simulink model "MAS_pc_up"  (R2022b)
settings: Solver=VariableStepAuto  StartTime=0.0  StopTime=300  RelTol=1e-3
values from neighbouring files (symbols this model uses):
  a1 = int8(3)    [init.m]
  A1 = [1.7,-1.3 ... (first row only)    [init.m]
  A2 = [1.8,-1.4 ... (first row only)    [init.m]
  a2 = int8(2)    [init.m]
  A3 = [1.4,-1.1 ... (first row only)    [init.m]
  a3 = int8(3)    [init.m]
  B1 = [1.0 ... (first row only)    [init.m]
  B2 = [1.7 ... (first row only)    [init.m]
  B3 = [0.8 ... (first row only)    [init.m]
  C1 = [1.0,0.3]    [init.m]
  C2 = [0.7,0.2]    [init.m]
  C3 = [1.1,0.4]    [init.m]
  F1 = [-0.4483 ... (first row only)    [init.m]
  F2 = [-0.6803 ... (first row only)    [init.m]
  F3 = [-0.3908 ... (first row only)    [init.m]
  G1 = -0.16    [init.m]
  G2 = -0.18    [init.m]
  G3 = -0.14    [init.m]
  H1 = -0.12    [init.m]
  H2 = -0.10    (= -0.1)    [init.m]
  H3 = -0.14    [init.m]
  M = [1,0,1 ... (first row only)    [init.m]
  s1 = int8(2)    [init.m]
  s2 = int8(3)    [init.m]
  s3 = int8(1)    [init.m]
  samp_t = 0.2    [init.m]
(part 2 of 2)

== system MAS_pc_up/u7 ==
  z : Inport
  hat_Y : Inport  Port=2
  Add : Sum
  Constant1 : Constant  Value=M
  Constant2 : Constant  Value=id
  G : Constant  Value=G1  VectorParams1D=off
  H : Constant  Value=H1  VectorParams1D=off
  MATLAB Function : MATLAB Function  TreatAsAtomicUnit=on
  Product : Product  Multiplication=Matrix(*)
  Product1 : Product  Multiplication=Matrix(*)
  u : Outport
  wires:
  z/1 -> Product/2
  G/1 -> Product/1
  Product/1 -> Add/1
  Add/1 -> u/1
  Constant1/1 -> MATLAB Function/1(M)
  hat_Y/1 -> MATLAB Function/2(hat_Y)
  Constant2/1 -> MATLAB Function/3(id)
  MATLAB Function/1(y) -> Product1/2
  H/1 -> Product1/1
  Product1/1 -> Add/2

== system MAS_pc_up/u8 ==
  z : Inport
  hat_Y : Inport  Port=2
  Add : Sum
  Constant1 : Constant  Value=M
  Constant2 : Constant  Value=id
  G : Constant  Value=G2  VectorParams1D=off
  H : Constant  Value=H2  VectorParams1D=off
  MATLAB Function : MATLAB Function  TreatAsAtomicUnit=on
  Product : Product  Multiplication=Matrix(*)
  Product1 : Product  Multiplication=Matrix(*)
  u : Outport
  wires:
  z/1 -> Product/2
  G/1 -> Product/1
  Product/1 -> Add/1
  Add/1 -> u/1
  Constant1/1 -> MATLAB Function/1(M)
  hat_Y/1 -> MATLAB Function/2(hat_Y)
  Constant2/1 -> MATLAB Function/3(id)
  MATLAB Function/1(y) -> Product1/2
  H/1 -> Product1/1
  Product1/1 -> Add/2

== system MAS_pc_up/u9 ==
  z : Inport
  hat_Y : Inport  Port=2
  Add : Sum
  Constant1 : Constant  Value=M
  Constant2 : Constant  Value=id
  G : Constant  Value=G3  VectorParams1D=off
  H : Constant  Value=H3  VectorParams1D=off
  MATLAB Function : MATLAB Function  TreatAsAtomicUnit=on
  Product : Product  Multiplication=Matrix(*)
  Product1 : Product  Multiplication=Matrix(*)
  u : Outport
  wires:
  z/1 -> Product/2
  G/1 -> Product/1
  Product/1 -> Add/1
  Add/1 -> u/1
  Constant1/1 -> MATLAB Function/1(M)
  hat_Y/1 -> MATLAB Function/2(hat_Y)
  Constant2/1 -> MATLAB Function/3(id)
  MATLAB Function/1(y) -> Product1/2
  H/1 -> Product1/1
  Product1/1 -> Add/2

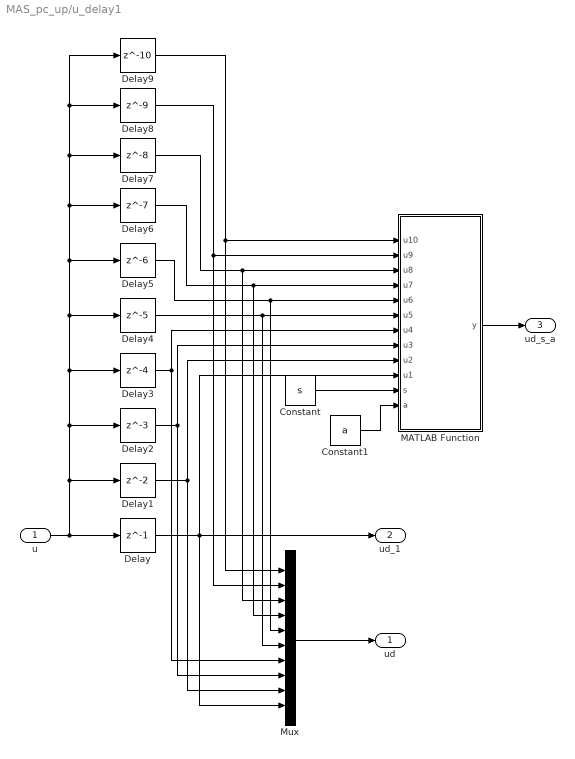
== system MAS_pc_up/u_delay1 ==
  u : Inport
  Constant : Constant  Value=s
  Constant1 : Constant  Value=a
  Delay : Delay  DelayLength=1  InitialCondition=0  SampleTime=samp_t
  Delay1 : Delay  InitialCondition=0  SampleTime=samp_t
  Delay2 : Delay  DelayLength=3  InitialCondition=0  SampleTime=samp_t
  Delay3 : Delay  DelayLength=4  InitialCondition=0  SampleTime=samp_t
  Delay4 : Delay  DelayLength=5  InitialCondition=0  SampleTime=samp_t
  Delay5 : Delay  DelayLength=6  InitialCondition=0  SampleTime=samp_t
  Delay6 : Delay  DelayLength=7  InitialCondition=0  SampleTime=samp_t
  Delay7 : Delay  DelayLength=8  InitialCondition=0  SampleTime=samp_t
  Delay8 : Delay  DelayLength=9  InitialCondition=0  SampleTime=samp_t
  Delay9 : Delay  DelayLength=10  InitialCondition=0  SampleTime=samp_t
  MATLAB Function : MATLAB Function  TreatAsAtomicUnit=on
  Mux : Mux  Inputs=10
  ud : Outport
  ud_1 : Outport  Port=2
  ud_s_a : Outport  Port=3
  wires:
  u/1 -> Delay/1, Delay1/1, Delay2/1, Delay3/1, Delay4/1, Delay6/1, Delay7/1, Delay8/1, Delay9/1, Delay5/1
  Delay/1 -> Mux/10, MATLAB Function/10(u1), ud_1/1
  Delay4/1 -> MATLAB Function/6(u5), Mux/6
  Delay3/1 -> Mux/7, MATLAB Function/7(u4)
  Delay2/1 -> Mux/8, MATLAB Function/8(u3)
  Delay1/1 -> Mux/9, MATLAB Function/9(u2)
  MATLAB Function/1(y) -> ud_s_a/1
  Mux/1 -> ud/1
  Delay5/1 -> Mux/5, MATLAB Function/5(u6)
  Delay6/1 -> MATLAB Function/4(u7), Mux/4
  Delay7/1 -> MATLAB Function/3(u8), Mux/3
  Delay8/1 -> MATLAB Function/2(u9), Mux/2
  Delay9/1 -> MATLAB Function/1(u10), Mux/1
  Constant/1 -> MATLAB Function/11(s)
  Constant1/1 -> MATLAB Function/12(a)

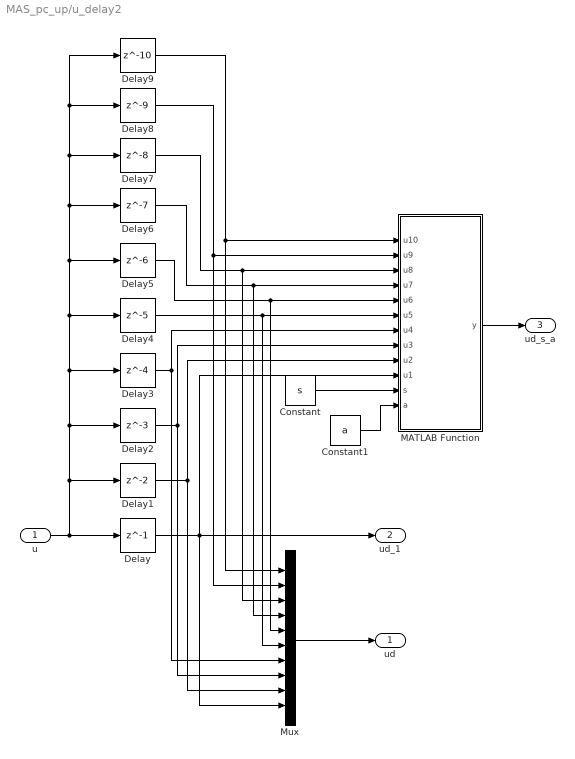
== system MAS_pc_up/u_delay2 ==
  u : Inport
  Constant : Constant  Value=s
  Constant1 : Constant  Value=a
  Delay : Delay  DelayLength=1  InitialCondition=0  SampleTime=samp_t
  Delay1 : Delay  InitialCondition=0  SampleTime=samp_t
  Delay2 : Delay  DelayLength=3  InitialCondition=0  SampleTime=samp_t
  Delay3 : Delay  DelayLength=4  InitialCondition=0  SampleTime=samp_t
  Delay4 : Delay  DelayLength=5  InitialCondition=0  SampleTime=samp_t
  Delay5 : Delay  DelayLength=6  InitialCondition=0  SampleTime=samp_t
  Delay6 : Delay  DelayLength=7  InitialCondition=0  SampleTime=samp_t
  Delay7 : Delay  DelayLength=8  InitialCondition=0  SampleTime=samp_t
  Delay8 : Delay  DelayLength=9  InitialCondition=0  SampleTime=samp_t
  Delay9 : Delay  DelayLength=10  InitialCondition=0  SampleTime=samp_t
  MATLAB Function : MATLAB Function  TreatAsAtomicUnit=on
  Mux : Mux  Inputs=10
  ud : Outport
  ud_1 : Outport  Port=2
  ud_s_a : Outport  Port=3
  wires:
  u/1 -> Delay/1, Delay1/1, Delay2/1, Delay3/1, Delay4/1, Delay6/1, Delay7/1, Delay8/1, Delay9/1, Delay5/1
  Delay/1 -> Mux/10, MATLAB Function/10(u1), ud_1/1
  Delay4/1 -> MATLAB Function/6(u5), Mux/6
  Delay3/1 -> Mux/7, MATLAB Function/7(u4)
  Delay2/1 -> Mux/8, MATLAB Function/8(u3)
  Delay1/1 -> Mux/9, MATLAB Function/9(u2)
  MATLAB Function/1(y) -> ud_s_a/1
  Mux/1 -> ud/1
  Delay5/1 -> Mux/5, MATLAB Function/5(u6)
  Delay6/1 -> MATLAB Function/4(u7), Mux/4
  Delay7/1 -> MATLAB Function/3(u8), Mux/3
  Delay8/1 -> MATLAB Function/2(u9), Mux/2
  Delay9/1 -> MATLAB Function/1(u10), Mux/1
  Constant/1 -> MATLAB Function/11(s)
  Constant1/1 -> MATLAB Function/12(a)

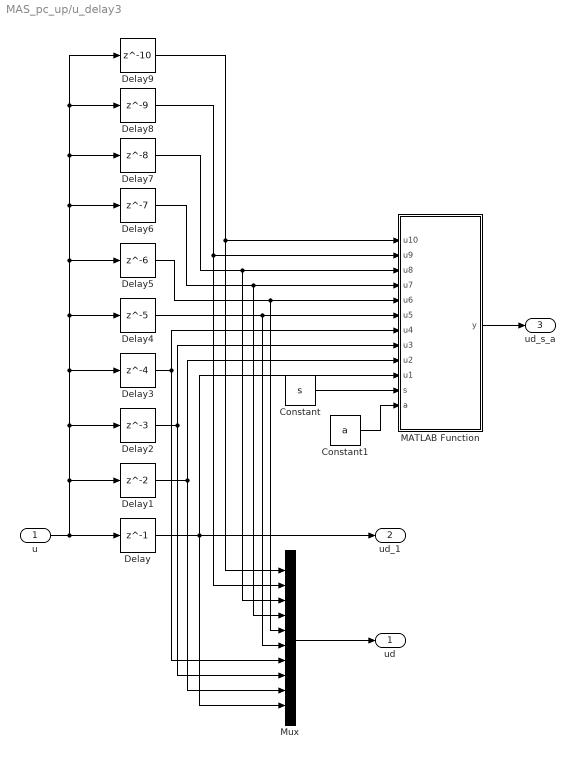
== system MAS_pc_up/u_delay3 ==
  u : Inport
  Constant : Constant  Value=s
  Constant1 : Constant  Value=a
  Delay : Delay  DelayLength=1  InitialCondition=0  SampleTime=samp_t
  Delay1 : Delay  InitialCondition=0  SampleTime=samp_t
  Delay2 : Delay  DelayLength=3  InitialCondition=0  SampleTime=samp_t
  Delay3 : Delay  DelayLength=4  InitialCondition=0  SampleTime=samp_t
  Delay4 : Delay  DelayLength=5  InitialCondition=0  SampleTime=samp_t
  Delay5 : Delay  DelayLength=6  InitialCondition=0  SampleTime=samp_t
  Delay6 : Delay  DelayLength=7  InitialCondition=0  SampleTime=samp_t
  Delay7 : Delay  DelayLength=8  InitialCondition=0  SampleTime=samp_t
  Delay8 : Delay  DelayLength=9  InitialCondition=0  SampleTime=samp_t
  Delay9 : Delay  DelayLength=10  InitialCondition=0  SampleTime=samp_t
  MATLAB Function : MATLAB Function  TreatAsAtomicUnit=on
  Mux : Mux  Inputs=10
  ud : Outport
  ud_1 : Outport  Port=2
  ud_s_a : Outport  Port=3
  wires:
  u/1 -> Delay/1, Delay1/1, Delay2/1, Delay3/1, Delay4/1, Delay6/1, Delay7/1, Delay8/1, Delay9/1, Delay5/1
  Delay/1 -> Mux/10, MATLAB Function/10(u1), ud_1/1
  Delay4/1 -> MATLAB Function/6(u5), Mux/6
  Delay3/1 -> Mux/7, MATLAB Function/7(u4)
  Delay2/1 -> Mux/8, MATLAB Function/8(u3)
  Delay1/1 -> Mux/9, MATLAB Function/9(u2)
  MATLAB Function/1(y) -> ud_s_a/1
  Mux/1 -> ud/1
  Delay5/1 -> Mux/5, MATLAB Function/5(u6)
  Delay6/1 -> MATLAB Function/4(u7), Mux/4
  Delay7/1 -> MATLAB Function/3(u8), Mux/3
  Delay8/1 -> MATLAB Function/2(u9), Mux/2
  Delay9/1 -> MATLAB Function/1(u10), Mux/1
  Constant/1 -> MATLAB Function/11(s)
  Constant1/1 -> MATLAB Function/12(a)

== system MAS_pc_up/u_delay4 ==
  u : Inport
  Constant : Constant  Value=s
  Delay : Delay  DelayLength=1  InitialCondition=0  SampleTime=samp_t
  Delay1 : Delay  InitialCondition=0  SampleTime=samp_t
  Delay2 : Delay  DelayLength=3  InitialCondition=0  SampleTime=samp_t
  Delay3 : Delay  DelayLength=4  InitialCondition=0  SampleTime=samp_t
  Delay4 : Delay  DelayLength=5  InitialCondition=0  SampleTime=samp_t
  MATLAB Function : MATLAB Function  TreatAsAtomicUnit=on
  Mux : Mux  Inputs=5
  ud : Outport
  ud_1 : Outport  Port=2
  ud_s : Outport  Port=3
  wires:
  u/1 -> Delay/1, Delay1/1, Delay2/1, Delay3/1, Delay4/1
  Delay/1 -> ud_1/1, MATLAB Function/6(u1), Mux/5
  Constant/1 -> MATLAB Function/1(s)
  Delay4/1 -> Mux/1, MATLAB Function/2(u5)
  Delay3/1 -> Mux/2, MATLAB Function/3(u4)
  Delay2/1 -> Mux/3, MATLAB Function/4(u3)
  Delay1/1 -> Mux/4, MATLAB Function/5(u2)
  MATLAB Function/1(y) -> ud_s/1
  Mux/1 -> ud/1

== system MAS_pc_up/u_delay5 ==
  u : Inport
  Constant : Constant  Value=s  OutDataTypeStr=int64
  Delay : Delay  DelayLength=1  InitialCondition=0  SampleTime=samp_t
  Delay1 : Delay  InitialCondition=0  SampleTime=samp_t
  Delay2 : Delay  DelayLength=3  InitialCondition=0  SampleTime=samp_t
  Delay3 : Delay  DelayLength=4  InitialCondition=0  SampleTime=samp_t
  Delay4 : Delay  DelayLength=5  InitialCondition=0  SampleTime=samp_t
  MATLAB Function : MATLAB Function  TreatAsAtomicUnit=on
  Mux : Mux  Inputs=5
  ud : Outport
  ud_1 : Outport  Port=2
  ud_s : Outport  Port=3
  wires:
  u/1 -> Delay/1, Delay1/1, Delay2/1, Delay3/1, Delay4/1
  Delay/1 -> ud_1/1, MATLAB Function/6(u1), Mux/5
  Constant/1 -> MATLAB Function/1(s)
  Delay4/1 -> Mux/1, MATLAB Function/2(u5)
  Delay3/1 -> Mux/2, MATLAB Function/3(u4)
  Delay2/1 -> Mux/3, MATLAB Function/4(u3)
  Delay1/1 -> Mux/4, MATLAB Function/5(u2)
  MATLAB Function/1(y) -> ud_s/1
  Mux/1 -> ud/1

== system MAS_pc_up/u_delay6 ==
  u : Inport
  Constant : Constant  Value=s
  Delay : Delay  DelayLength=1  InitialCondition=0  SampleTime=samp_t
  Delay1 : Delay  InitialCondition=0  SampleTime=samp_t
  Delay2 : Delay  DelayLength=3  InitialCondition=0  SampleTime=samp_t
  Delay3 : Delay  DelayLength=4  InitialCondition=0  SampleTime=samp_t
  Delay4 : Delay  DelayLength=5  InitialCondition=0  SampleTime=samp_t
  MATLAB Function : MATLAB Function  TreatAsAtomicUnit=on
  Mux : Mux  Inputs=5
  ud : Outport
  ud_1 : Outport  Port=2
  ud_s : Outport  Port=3
  wires:
  u/1 -> Delay/1, Delay1/1, Delay2/1, Delay3/1, Delay4/1
  Delay/1 -> ud_1/1, MATLAB Function/6(u1), Mux/5
  Constant/1 -> MATLAB Function/1(s)
  Delay4/1 -> Mux/1, MATLAB Function/2(u5)
  Delay3/1 -> Mux/2, MATLAB Function/3(u4)
  Delay2/1 -> Mux/3, MATLAB Function/4(u3)
  Delay1/1 -> Mux/4, MATLAB Function/5(u2)
  MATLAB Function/1(y) -> ud_s/1
  Mux/1 -> ud/1

== matlab function MAS_pc_up/u2/MATLAB Function ==
  data: M input; y output; hat_Y input; id input
function y = fcn(M,hat_Y,id)
y = zeros(size(hat_Y(id,:)))
for i = 1:length(M(id,:))
    if M(id,i)==1
        y = y + hat_Y(i,:) - hat_Y(id,:)
    end

end

== matlab function MAS_pc_up/u3/MATLAB Function ==
  data: M input; y output; hat_Y input; id input
function y = fcn(M,hat_Y,id)
y = zeros(size(hat_Y(id,:)))
for i = 1:length(M(id,:))
    if M(id,i)==1
        y = y + hat_Y(i,:) - hat_Y(id,:)
    end

end

== matlab function MAS_pc_up/u_delay1/MATLAB Function ==
  data: u10 input; u9 input; u8 input; u7 input; u6 input; y output size=1*1; u5 input size=1*1; u4 input size=1*1; u3 input size=1*1; u2 input size=1*1; u1 input size=1*1; s input; a input
function y = fcn(u10,u9,u8,u7,u6,u5,u4,u3,u2,u1,s,a)
tmp = s + a;
if tmp==1
    y = u1;
elseif tmp==2
    y = u2;
elseif tmp==3
    y = u3;
elseif tmp==4
    y = u4;
elseif tmp==5
    y = u5;
elseif tmp==6
    y = u6;
elseif tmp==7
    y = u7;
elseif tmp==8
    y = u8;
elseif tmp==9
    y = u9;
elseif tmp==10
    y = u10;
else
    y = u1
disp("mmp_error")
end

== matlab function MAS_pc_up/u_delay2/MATLAB Function ==
  data: u10 input; u9 input; u8 input; u7 input; u6 input; y output size=1*1; u5 input size=1*1; u4 input size=1*1; u3 input size=1*1; u2 input size=1*1; u1 input size=1*1; s input; a input
function y = fcn(u10,u9,u8,u7,u6,u5,u4,u3,u2,u1,s,a)
tmp = s + a;
if tmp==1
    y = u1;
elseif tmp==2
    y = u2;
elseif tmp==3
    y = u3;
elseif tmp==4
    y = u4;
elseif tmp==5
    y = u5;
elseif tmp==6
    y = u6;
elseif tmp==7
    y = u7;
elseif tmp==8
    y = u8;
elseif tmp==9
    y = u9;
elseif tmp==10
    y = u10;
else
    y = u1
disp("mmp_error")
end

== matlab function MAS_pc_up/u_delay3/MATLAB Function ==
  data: u10 input; u9 input; u8 input; u7 input; u6 input; y output size=1*1; u5 input size=1*1; u4 input size=1*1; u3 input size=1*1; u2 input size=1*1; u1 input size=1*1; s input; a input
function y = fcn(u10,u9,u8,u7,u6,u5,u4,u3,u2,u1,s,a)
tmp = s + a;
if tmp==1
    y = u1;
elseif tmp==2
    y = u2;
elseif tmp==3
    y = u3;
elseif tmp==4
    y = u4;
elseif tmp==5
    y = u5;
elseif tmp==6
    y = u6;
elseif tmp==7
    y = u7;
elseif tmp==8
    y = u8;
elseif tmp==9
    y = u9;
elseif tmp==10
    y = u10;
else
    y = u1
disp("mmp_error")
end

== matlab function MAS_pc_up/Ps2a2/MATLAB Function ==
  data: u10 input; u9 input; u8 input; u7 input; u6 input; x_ output size=2*1; u5 input; u4 input; u3 input; u2 input; u1 input; y output size=1*1; x input size=2*1; s input; a input; A input; B input; C input
function [x_,y]= fcn(u10,u9,u8,u7,u6,u5,u4,u3,u2,u1,x,s,a,A,B,C)
% tau的上界是N,最多迭代N次，控制输入按照t-s_i时刻的值
tau = s + a;
temp0 = x;
if tau == 1
    temp1 = A * temp0 + B * u1;
    x_ = temp1;
elseif tau == 2
    temp1 = A * temp0 + B * u2;
    temp2 = A * temp1 + B * u1;
    x_ = temp2;
elseif tau == 3
    temp1 = A * temp0 + B * u3;
    temp2 = A * temp1 + B * u2;
    temp3 = A * temp2 + B * u1;
    x_ = temp3;
elseif tau == 4
    temp1 = A * temp0 + B * u4;
    temp2 = A * temp1 + B * u3;
    temp3 = A * temp2 + B * u2;
    temp4 = A * temp3 + B * u1;
    x_ = temp4;  
elseif tau == 5
    temp1 = A * temp0 + B * u5;
    temp2 = A * temp1 + B * u4;
    temp3 = A * temp2 + B * u3;
    temp4 = A * temp3 + B * u2;
    temp5 = A * temp4 + B * u1;
    x_ = temp5;
elseif tau == 6
    temp1 = A * temp0 + B * u6;
    temp2 = A * temp1 + B * u5;
    temp3 = A * temp2 + B * u4;
    temp4 = A * temp3 + B * u3;
    temp5 = A * temp4 + B * u2;
    temp6 = A * temp5 + B * u1;
    x_ = temp6;
elseif tau == 7
    temp1 = A * temp0 + B * u7;
    temp2 = A * temp1 + B * u6;
    temp3 = A * temp2 + B * u5;
    temp4 = A * temp3 + B * u4;
    temp5 = A * temp4 + B * u3;
    temp6 = A * temp5 + B * u2;
    temp7 = A * temp6 + B * u2;
    x_ = temp7;
elseif tau == 8
    temp1 = A * temp0 + B * u8;
    temp2 = A * temp1 + B * u7;
    temp3 = A * temp2 + B * u6;
    temp4 = A * temp3 + B * u5;
    temp5 = A * temp4 + B * u4;
    temp6 = A * temp5 + B * u3;
    temp7 = A * temp6 + B * u2;
    temp8 = A * temp7 + B * u1;
    x_ = temp8;
elseif tau == 9
    temp1 = A * temp0 + B * u9;
    temp2 = A * temp1 + B * u8;
    temp3 = A * temp2 + B * u7;
    temp4 = A * temp3 + B * u6;
    temp5 = A * temp4 + B * u5;
    temp6 = A * temp5 + B * u4;
    temp7 = A * temp6 + B * u3;
    temp8 = A * temp7 + B * u2;
    temp9 = A * temp8 + B * u1;
    x_ = temp9;
elseif tau == 10
    temp1 = A * temp0 + B * u10;
    temp2 = A * temp1 + B * u9;
    temp3 = A * temp2 + B * u8;
    temp4 = A * temp3 + B * u7;
    temp5 = A * temp4 + B * u6;
    temp6 = A * temp5 + B * u5;
    temp7 = A * temp6 + B * u4;
    temp8 = A * temp7 + B * u3;
    temp9 = A * temp8 + B * u2;
    temp10 = A * temp9 + B * u1;
    x_ = temp10;
else 
    x_ = temp0;

end
y = C * x_;

== matlab function MAS_pc_up/Ps2a1/MATLAB Function ==
  data: u10 input; u9 input; u8 input; u7 input; u6 input; x_ output size=2*1; u5 input; u4 input; u3 input; u2 input; u1 input; y output size=1*1; x input size=2*1; s input; a input; A input; B input; C input
function [x_,y]= fcn(u10,u9,u8,u7,u6,u5,u4,u3,u2,u1,x,s,a,A,B,C)
% tau的上界是N,最多迭代N次，控制输入按照t-s_i时刻的值
tau = s + a;
temp0 = x;
if tau == 1
    temp1 = A * temp0 + B * u1;
    x_ = temp1;
elseif tau == 2
    temp1 = A * temp0 + B * u2;
    temp2 = A * temp1 + B * u1;
    x_ = temp2;
elseif tau == 3
    temp1 = A * temp0 + B * u3;
    temp2 = A * temp1 + B * u2;
    temp3 = A * temp2 + B * u1;
    x_ = temp3;
elseif tau == 4
    temp1 = A * temp0 + B * u4;
    temp2 = A * temp1 + B * u3;
    temp3 = A * temp2 + B * u2;
    temp4 = A * temp3 + B * u1;
    x_ = temp4;  
elseif tau == 5
    temp1 = A * temp0 + B * u5;
    temp2 = A * temp1 + B * u4;
    temp3 = A * temp2 + B * u3;
    temp4 = A * temp3 + B * u2;
    temp5 = A * temp4 + B * u1;
    x_ = temp5;
elseif tau == 6
    temp1 = A * temp0 + B * u6;
    temp2 = A * temp1 + B * u5;
    temp3 = A * temp2 + B * u4;
    temp4 = A * temp3 + B * u3;
    temp5 = A * temp4 + B * u2;
    temp6 = A * temp5 + B * u1;
    x_ = temp6;
elseif tau == 7
    temp1 = A * temp0 + B * u7;
    temp2 = A * temp1 + B * u6;
    temp3 = A * temp2 + B * u5;
    temp4 = A * temp3 + B * u4;
    temp5 = A * temp4 + B * u3;
    temp6 = A * temp5 + B * u2;
    temp7 = A * temp6 + B * u2;
    x_ = temp7;
elseif tau == 8
    temp1 = A * temp0 + B * u8;
    temp2 = A * temp1 + B * u7;
    temp3 = A * temp2 + B * u6;
    temp4 = A * temp3 + B * u5;
    temp5 = A * temp4 + B * u4;
    temp6 = A * temp5 + B * u3;
    temp7 = A * temp6 + B * u2;
    temp8 = A * temp7 + B * u1;
    x_ = temp8;
elseif tau == 9
    temp1 = A * temp0 + B * u9;
    temp2 = A * temp1 + B * u8;
    temp3 = A * temp2 + B * u7;
    temp4 = A * temp3 + B * u6;
    temp5 = A * temp4 + B * u5;
    temp6 = A * temp5 + B * u4;
    temp7 = A * temp6 + B * u3;
    temp8 = A * temp7 + B * u2;
    temp9 = A * temp8 + B * u1;
    x_ = temp9;
elseif tau == 10
    temp1 = A * temp0 + B * u10;
    temp2 = A * temp1 + B * u9;
    temp3 = A * temp2 + B * u8;
    temp4 = A * temp3 + B * u7;
    temp5 = A * temp4 + B * u6;
    temp6 = A * temp5 + B * u5;
    temp7 = A * temp6 + B * u4;
    temp8 = A * temp7 + B * u3;
    temp9 = A * temp8 + B * u2;
    temp10 = A * temp9 + B * u1;
    x_ = temp10;
else 
    x_ = temp0;

end
y = C * x_;

== matlab function MAS_pc_up/Ps2a3/MATLAB Function ==
  data: u10 input; u9 input; u8 input; u7 input; u6 input; x_ output size=2*1; u5 input; u4 input; u3 input; u2 input; u1 input; y output size=1*1; x input size=2*1; s input; a input; A input; B input; C input
function [x_,y]= fcn(u10,u9,u8,u7,u6,u5,u4,u3,u2,u1,x,s,a,A,B,C)
% tau的上界是N,最多迭代N次，控制输入按照t-s_i时刻的值
tau = s + a;
temp0 = x;
if tau == 1
    temp1 = A * temp0 + B * u1;
    x_ = temp1;
elseif tau == 2
    temp1 = A * temp0 + B * u2;
    temp2 = A * temp1 + B * u1;
    x_ = temp2;
elseif tau == 3
    temp1 = A * temp0 + B * u3;
    temp2 = A * temp1 + B * u2;
    temp3 = A * temp2 + B * u1;
    x_ = temp3;
elseif tau == 4
    temp1 = A * temp0 + B * u4;
    temp2 = A * temp1 + B * u3;
    temp3 = A * temp2 + B * u2;
    temp4 = A * temp3 + B * u1;
    x_ = temp4;  
elseif tau == 5
    temp1 = A * temp0 + B * u5;
    temp2 = A * temp1 + B * u4;
    temp3 = A * temp2 + B * u3;
    temp4 = A * temp3 + B * u2;
    temp5 = A * temp4 + B * u1;
    x_ = temp5;
elseif tau == 6
    temp1 = A * temp0 + B * u6;
    temp2 = A * temp1 + B * u5;
    temp3 = A * temp2 + B * u4;
    temp4 = A * temp3 + B * u3;
    temp5 = A * temp4 + B * u2;
    temp6 = A * temp5 + B * u1;
    x_ = temp6;
elseif tau == 7
    temp1 = A * temp0 + B * u7;
    temp2 = A * temp1 + B * u6;
    temp3 = A * temp2 + B * u5;
    temp4 = A * temp3 + B * u4;
    temp5 = A * temp4 + B * u3;
    temp6 = A * temp5 + B * u2;
    temp7 = A * temp6 + B * u2;
    x_ = temp7;
elseif tau == 8
    temp1 = A * temp0 + B * u8;
    temp2 = A * temp1 + B * u7;
    temp3 = A * temp2 + B * u6;
    temp4 = A * temp3 + B * u5;
    temp5 = A * temp4 + B * u4;
    temp6 = A * temp5 + B * u3;
    temp7 = A * temp6 + B * u2;
    temp8 = A * temp7 + B * u1;
    x_ = temp8;
elseif tau == 9
    temp1 = A * temp0 + B * u9;
    temp2 = A * temp1 + B * u8;
    temp3 = A * temp2 + B * u7;
    temp4 = A * temp3 + B * u6;
    temp5 = A * temp4 + B * u5;
    temp6 = A * temp5 + B * u4;
    temp7 = A * temp6 + B * u3;
    temp8 = A * temp7 + B * u2;
    temp9 = A * temp8 + B * u1;
    x_ = temp9;
elseif tau == 10
    temp1 = A * temp0 + B * u10;
    temp2 = A * temp1 + B * u9;
    temp3 = A * temp2 + B * u8;
    temp4 = A * temp3 + B * u7;
    temp5 = A * temp4 + B * u6;
    temp6 = A * temp5 + B * u5;
    temp7 = A * temp6 + B * u4;
    temp8 = A * temp7 + B * u3;
    temp9 = A * temp8 + B * u2;
    temp10 = A * temp9 + B * u1;
    x_ = temp10;
else 
    x_ = temp0;

end
y = C * x_;

== matlab function MAS_pc_up/MATLAB Function2 ==
  data: t input; r output
function r = fcn(t)
if t<100
    r = 1;
elseif t<200
    r = 0;

elseif t<300
    r = 1;
else 
    r = 0;

end

== matlab function MAS_pc_up/Ps3a3/MATLAB Function ==
  data: u10 input; u9 input; u8 input; u7 input; u6 input; x_ output size=2*1; u5 input; u4 input; u3 input; u2 input; u1 input; y output size=1*1; x input size=2*1; s input; a input; A input; B input; C input
function [x_,y]= fcn(u10,u9,u8,u7,u6,u5,u4,u3,u2,u1,x,s,a,A,B,C)
% tau的上界是N,最多迭代N次，控制输入按照t-s_i时刻的值
tau = s + a;
temp0 = x;
if tau == 1
    temp1 = A * temp0 + B * u1;
    x_ = temp1;
elseif tau == 2
    temp1 = A * temp0 + B * u2;
    temp2 = A * temp1 + B * u1;
    x_ = temp2;
elseif tau == 3
    temp1 = A * temp0 + B * u3;
    temp2 = A * temp1 + B * u2;
    temp3 = A * temp2 + B * u1;
    x_ = temp3;
elseif tau == 4
    temp1 = A * temp0 + B * u4;
    temp2 = A * temp1 + B * u3;
    temp3 = A * temp2 + B * u2;
    temp4 = A * temp3 + B * u1;
    x_ = temp4;  
elseif tau == 5
    temp1 = A * temp0 + B * u5;
    temp2 = A * temp1 + B * u4;
    temp3 = A * temp2 + B * u3;
    temp4 = A * temp3 + B * u2;
    temp5 = A * temp4 + B * u1;
    x_ = temp5;
elseif tau == 6
    temp1 = A * temp0 + B * u6;
    temp2 = A * temp1 + B * u5;
    temp3 = A * temp2 + B * u4;
    temp4 = A * temp3 + B * u3;
    temp5 = A * temp4 + B * u2;
    temp6 = A * temp5 + B * u1;
    x_ = temp6;
elseif tau == 7
    temp1 = A * temp0 + B * u7;
    temp2 = A * temp1 + B * u6;
    temp3 = A * temp2 + B * u5;
    temp4 = A * temp3 + B * u4;
    temp5 = A * temp4 + B * u3;
    temp6 = A * temp5 + B * u2;
    temp7 = A * temp6 + B * u2;
    x_ = temp7;
elseif tau == 8
    temp1 = A * temp0 + B * u8;
    temp2 = A * temp1 + B * u7;
    temp3 = A * temp2 + B * u6;
    temp4 = A * temp3 + B * u5;
    temp5 = A * temp4 + B * u4;
    temp6 = A * temp5 + B * u3;
    temp7 = A * temp6 + B * u2;
    temp8 = A * temp7 + B * u1;
    x_ = temp8;
elseif tau == 9
    temp1 = A * temp0 + B * u9;
    temp2 = A * temp1 + B * u8;
    temp3 = A * temp2 + B * u7;
    temp4 = A * temp3 + B * u6;
    temp5 = A * temp4 + B * u5;
    temp6 = A * temp5 + B * u4;
    temp7 = A * temp6 + B * u3;
    temp8 = A * temp7 + B * u2;
    temp9 = A * temp8 + B * u1;
    x_ = temp9;
elseif tau == 10
    temp1 = A * temp0 + B * u10;
    temp2 = A * temp1 + B * u9;
    temp3 = A * temp2 + B * u8;
    temp4 = A * temp3 + B * u7;
    temp5 = A * temp4 + B * u6;
    temp6 = A * temp5 + B * u5;
    temp7 = A * temp6 + B * u4;
    temp8 = A * temp7 + B * u3;
    temp9 = A * temp8 + B * u2;
    temp10 = A * temp9 + B * u1;
    x_ = temp10;
else 
    x_ = temp0;

end
y = C * x_;

== matlab function MAS_pc_up/Ps3a1/MATLAB Function ==
  data: u10 input; u9 input; u8 input; u7 input; u6 input; x_ output size=2*1; u5 input; u4 input; u3 input; u2 input; u1 input; y output size=1*1; x input size=2*1; s input; a input; A input; B input; C input
function [x_,y]= fcn(u10,u9,u8,u7,u6,u5,u4,u3,u2,u1,x,s,a,A,B,C)
% tau的上界是N,最多迭代N次，控制输入按照t-s_i时刻的值
tau = s + a;
temp0 = x;
if tau == 1
    temp1 = A * temp0 + B * u1;
    x_ = temp1;
elseif tau == 2
    temp1 = A * temp0 + B * u2;
    temp2 = A * temp1 + B * u1;
    x_ = temp2;
elseif tau == 3
    temp1 = A * temp0 + B * u3;
    temp2 = A * temp1 + B * u2;
    temp3 = A * temp2 + B * u1;
    x_ = temp3;
elseif tau == 4
    temp1 = A * temp0 + B * u4;
    temp2 = A * temp1 + B * u3;
    temp3 = A * temp2 + B * u2;
    temp4 = A * temp3 + B * u1;
    x_ = temp4;  
elseif tau == 5
    temp1 = A * temp0 + B * u5;
    temp2 = A * temp1 + B * u4;
    temp3 = A * temp2 + B * u3;
    temp4 = A * temp3 + B * u2;
    temp5 = A * temp4 + B * u1;
    x_ = temp5;
elseif tau == 6
    temp1 = A * temp0 + B * u6;
    temp2 = A * temp1 + B * u5;
    temp3 = A * temp2 + B * u4;
    temp4 = A * temp3 + B * u3;
    temp5 = A * temp4 + B * u2;
    temp6 = A * temp5 + B * u1;
    x_ = temp6;
elseif tau == 7
    temp1 = A * temp0 + B * u7;
    temp2 = A * temp1 + B * u6;
    temp3 = A * temp2 + B * u5;
    temp4 = A * temp3 + B * u4;
    temp5 = A * temp4 + B * u3;
    temp6 = A * temp5 + B * u2;
    temp7 = A * temp6 + B * u2;
    x_ = temp7;
elseif tau == 8
    temp1 = A * temp0 + B * u8;
    temp2 = A * temp1 + B * u7;
    temp3 = A * temp2 + B * u6;
    temp4 = A * temp3 + B * u5;
    temp5 = A * temp4 + B * u4;
    temp6 = A * temp5 + B * u3;
    temp7 = A * temp6 + B * u2;
    temp8 = A * temp7 + B * u1;
    x_ = temp8;
elseif tau == 9
    temp1 = A * temp0 + B * u9;
    temp2 = A * temp1 + B * u8;
    temp3 = A * temp2 + B * u7;
    temp4 = A * temp3 + B * u6;
    temp5 = A * temp4 + B * u5;
    temp6 = A * temp5 + B * u4;
    temp7 = A * temp6 + B * u3;
    temp8 = A * temp7 + B * u2;
    temp9 = A * temp8 + B * u1;
    x_ = temp9;
elseif tau == 10
    temp1 = A * temp0 + B * u10;
    temp2 = A * temp1 + B * u9;
    temp3 = A * temp2 + B * u8;
    temp4 = A * temp3 + B * u7;
    temp5 = A * temp4 + B * u6;
    temp6 = A * temp5 + B * u5;
    temp7 = A * temp6 + B * u4;
    temp8 = A * temp7 + B * u3;
    temp9 = A * temp8 + B * u2;
    temp10 = A * temp9 + B * u1;
    x_ = temp10;
else 
    x_ = temp0;

end
y = C * x_;

== matlab function MAS_pc_up/Ps3a2/MATLAB Function ==
  data: u10 input; u9 input; u8 input; u7 input; u6 input; x_ output size=2*1; u5 input; u4 input; u3 input; u2 input; u1 input; y output size=1*1; x input size=2*1; s input; a input; A input; B input; C input
function [x_,y]= fcn(u10,u9,u8,u7,u6,u5,u4,u3,u2,u1,x,s,a,A,B,C)
% tau的上界是N,最多迭代N次，控制输入按照t-s_i时刻的值
tau = s + a;
temp0 = x;
if tau == 1
    temp1 = A * temp0 + B * u1;
    x_ = temp1;
elseif tau == 2
    temp1 = A * temp0 + B * u2;
    temp2 = A * temp1 + B * u1;
    x_ = temp2;
elseif tau == 3
    temp1 = A * temp0 + B * u3;
    temp2 = A * temp1 + B * u2;
    temp3 = A * temp2 + B * u1;
    x_ = temp3;
elseif tau == 4
    temp1 = A * temp0 + B * u4;
    temp2 = A * temp1 + B * u3;
    temp3 = A * temp2 + B * u2;
    temp4 = A * temp3 + B * u1;
    x_ = temp4;  
elseif tau == 5
    temp1 = A * temp0 + B * u5;
    temp2 = A * temp1 + B * u4;
    temp3 = A * temp2 + B * u3;
    temp4 = A * temp3 + B * u2;
    temp5 = A * temp4 + B * u1;
    x_ = temp5;
elseif tau == 6
    temp1 = A * temp0 + B * u6;
    temp2 = A * temp1 + B * u5;
    temp3 = A * temp2 + B * u4;
    temp4 = A * temp3 + B * u3;
    temp5 = A * temp4 + B * u2;
    temp6 = A * temp5 + B * u1;
    x_ = temp6;
elseif tau == 7
    temp1 = A * temp0 + B * u7;
    temp2 = A * temp1 + B * u6;
    temp3 = A * temp2 + B * u5;
    temp4 = A * temp3 + B * u4;
    temp5 = A * temp4 + B * u3;
    temp6 = A * temp5 + B * u2;
    temp7 = A * temp6 + B * u2;
    x_ = temp7;
elseif tau == 8
    temp1 = A * temp0 + B * u8;
    temp2 = A * temp1 + B * u7;
    temp3 = A * temp2 + B * u6;
    temp4 = A * temp3 + B * u5;
    temp5 = A * temp4 + B * u4;
    temp6 = A * temp5 + B * u3;
    temp7 = A * temp6 + B * u2;
    temp8 = A * temp7 + B * u1;
    x_ = temp8;
elseif tau == 9
    temp1 = A * temp0 + B * u9;
    temp2 = A * temp1 + B * u8;
    temp3 = A * temp2 + B * u7;
    temp4 = A * temp3 + B * u6;
    temp5 = A * temp4 + B * u5;
    temp6 = A * temp5 + B * u4;
    temp7 = A * temp6 + B * u3;
    temp8 = A * temp7 + B * u2;
    temp9 = A * temp8 + B * u1;
    x_ = temp9;
elseif tau == 10
    temp1 = A * temp0 + B * u10;
    temp2 = A * temp1 + B * u9;
    temp3 = A * temp2 + B * u8;
    temp4 = A * temp3 + B * u7;
    temp5 = A * temp4 + B * u6;
    temp6 = A * temp5 + B * u5;
    temp7 = A * temp6 + B * u4;
    temp8 = A * temp7 + B * u3;
    temp9 = A * temp8 + B * u2;
    temp10 = A * temp9 + B * u1;
    x_ = temp10;
else 
    x_ = temp0;

end
y = C * x_;

== matlab function MAS_pc_up/Ps1a1/MATLAB Function ==
  data: u10 input; u9 input; u8 input; u7 input; u6 input; x_ output size=2*1; u5 input; u4 input; u3 input; u2 input; u1 input; y output size=1*1; x input size=2*1; s input; a input; A input; B input; C input
function [x_,y]= fcn(u10,u9,u8,u7,u6,u5,u4,u3,u2,u1,x,s,a,A,B,C)
% tau的上界是N,最多迭代N次，控制输入按照t-s_i时刻的值
tau = s + a;
temp0 = x;
if tau == 1
    temp1 = A * temp0 + B * u1;
    x_ = temp1;
elseif tau == 2
    temp1 = A * temp0 + B * u2;
    temp2 = A * temp1 + B * u1;
    x_ = temp2;
elseif tau == 3
    temp1 = A * temp0 + B * u3;
    temp2 = A * temp1 + B * u2;
    temp3 = A * temp2 + B * u1;
    x_ = temp3;
elseif tau == 4
    temp1 = A * temp0 + B * u4;
    temp2 = A * temp1 + B * u3;
    temp3 = A * temp2 + B * u2;
    temp4 = A * temp3 + B * u1;
    x_ = temp4;  
elseif tau == 5
    temp1 = A * temp0 + B * u5;
    temp2 = A * temp1 + B * u4;
    temp3 = A * temp2 + B * u3;
    temp4 = A * temp3 + B * u2;
    temp5 = A * temp4 + B * u1;
    x_ = temp5;
elseif tau == 6
    temp1 = A * temp0 + B * u6;
    temp2 = A * temp1 + B * u5;
    temp3 = A * temp2 + B * u4;
    temp4 = A * temp3 + B * u3;
    temp5 = A * temp4 + B * u2;
    temp6 = A * temp5 + B * u1;
    x_ = temp6;
elseif tau == 7
    temp1 = A * temp0 + B * u7;
    temp2 = A * temp1 + B * u6;
    temp3 = A * temp2 + B * u5;
    temp4 = A * temp3 + B * u4;
    temp5 = A * temp4 + B * u3;
    temp6 = A * temp5 + B * u2;
    temp7 = A * temp6 + B * u2;
    x_ = temp7;
elseif tau == 8
    temp1 = A * temp0 + B * u8;
    temp2 = A * temp1 + B * u7;
    temp3 = A * temp2 + B * u6;
    temp4 = A * temp3 + B * u5;
    temp5 = A * temp4 + B * u4;
    temp6 = A * temp5 + B * u3;
    temp7 = A * temp6 + B * u2;
    temp8 = A * temp7 + B * u1;
    x_ = temp8;
elseif tau == 9
    temp1 = A * temp0 + B * u9;
    temp2 = A * temp1 + B * u8;
    temp3 = A * temp2 + B * u7;
    temp4 = A * temp3 + B * u6;
    temp5 = A * temp4 + B * u5;
    temp6 = A * temp5 + B * u4;
    temp7 = A * temp6 + B * u3;
    temp8 = A * temp7 + B * u2;
    temp9 = A * temp8 + B * u1;
    x_ = temp9;
elseif tau == 10
    temp1 = A * temp0 + B * u10;
    temp2 = A * temp1 + B * u9;
    temp3 = A * temp2 + B * u8;
    temp4 = A * temp3 + B * u7;
    temp5 = A * temp4 + B * u6;
    temp6 = A * temp5 + B * u5;
    temp7 = A * temp6 + B * u4;
    temp8 = A * temp7 + B * u3;
    temp9 = A * temp8 + B * u2;
    temp10 = A * temp9 + B * u1;
    x_ = temp10;
else 
    x_ = temp0;

end
y = C * x_;

== matlab function MAS_pc_up/MATLAB Function1 ==
  data: t input; r output
function r = fcn(t)
if t<100
    r = 1;
elseif t<200
    r = 0;

elseif t<300
    r = 1;
else 
    r = 0;

end

== matlab function MAS_pc_up/MATLAB Function3 ==
  data: t input; r output
function r = fcn(t)
if t<100
    r = 1;
elseif t<200
    r = 0;

elseif t<300
    r = 1;
else 
    r = 0;

end

== matlab function MAS_pc_up/u7/MATLAB Function ==
  data: M input; y output; hat_Y input; id input
function y = fcn(M,hat_Y,id)
y = zeros(size(hat_Y(id,:)))
for i = 1:length(M(id,:))
    if M(id,i)==1
        y = y + hat_Y(i,:) - hat_Y(id,:);
    end

end

== matlab function MAS_pc_up/u8/MATLAB Function ==
  data: M input; y output; hat_Y input; id input
function y = fcn(M,hat_Y,id)
y = zeros(size(hat_Y(id,:)))
for i = 1:length(M(id,:))
    if M(id,i)==1
        y = y + hat_Y(i,:) - hat_Y(id,:)
    end

end

== matlab function MAS_pc_up/u9/MATLAB Function ==
  data: M input; y output; hat_Y input; id input
function y = fcn(M,hat_Y,id)
y = zeros(size(hat_Y(id,:)))
for i = 1:length(M(id,:))
    if M(id,i)==1
        y = y + hat_Y(i,:) - hat_Y(id,:)
    end

end

== matlab function MAS_pc_up/MATLAB Function ==
  data: t input; r output
function r = fcn(t)
if t<100
    r = 1;
elseif t<200
    r = 0;

elseif t<300
    r = 1;
else 
    r = 0;

end

== matlab function MAS_pc_up/u10/MATLAB Function ==
  data: M input; y output; hat_Y input; id input
function y = fcn(M,hat_Y,id)
y = zeros(size(hat_Y(id,:)))
for i = 1:length(M(id,:))
    if M(id,i)==1
        y = y + hat_Y(i,:) - hat_Y(id,:);
    end

end

== matlab function MAS_pc_up/u11/MATLAB Function ==
  data: M input; y output; hat_Y input; id input
function y = fcn(M,hat_Y,id)
y = zeros(size(hat_Y(id,:)))
for i = 1:length(M(id,:))
    if M(id,i)==1
        y = y + hat_Y(i,:) - hat_Y(id,:)
    end

end

== matlab function MAS_pc_up/u12/MATLAB Function ==
  data: M input; y output; hat_Y input; id input
function y = fcn(M,hat_Y,id)
y = zeros(size(hat_Y(id,:)))
for i = 1:length(M(id,:))
    if M(id,i)==1
        y = y + hat_Y(i,:) - hat_Y(id,:)
    end

end

== matlab function MAS_pc_up/Ps4/MATLAB Function ==
  data: x_ output size=2*1; u5 input; u4 input; u3 input; u2 input; u1 input; y output size=1*1; x input size=2*1; tau input; A input; B input; C input
function [x_,y]= fcn(u5,u4,u3,u2,u1,x,tau,A,B,C)
% tau的上界是N,最多迭代N次，控制输入按照t-s_i时刻的值
temp0 = x;
if tau == 1
    temp1 = A * x + B * u1;
    x_ = temp1;
elseif tau == 2
    temp1 = A * x + B * u2;
    temp2 = A * temp1 + B * u1;
    x_ = temp2;
elseif tau == 3
    temp1 = A * x + B * u3;
    temp2 = A * temp1 + B * u2;
    temp3 = A * temp2 + B * u1;
    x_ = temp3;
elseif tau == 4
    temp1 = A * x + B * u4;
    temp2 = A * temp1 + B * u3;
    temp3 = A * temp2 + B * u2;
    temp4 = A * temp3 + B * u1;
    x_ = temp4;
    
elseif tau == 5
    temp1 = A * x + B * u5;
    temp2 = A * temp1 + B * u4;
    temp3 = A * temp2 + B * u3;
    temp4 = A * temp3 + B * u2;
    temp5 = A * temp4 + B * u1;
    x_ = temp5;
else 
    x_ = temp0;
end
y = C * x_;

== matlab function MAS_pc_up/Ps5/MATLAB Function ==
  data: x_ output size=2*1; u5 input; u4 input; u3 input; u2 input; u1 input; y output size=1*1; x input size=2*1; tau input; A input; B input; C input
function [x_,y]= fcn(u5,u4,u3,u2,u1,x,tau,A,B,C)
% tau的上界是N,最多迭代N次，控制输入按照t-s_i时刻的值
temp0 = x;
if tau == 1
    temp1 = A * x + B * u1;
    x_ = temp1;
elseif tau == 2
    temp1 = A * x + B * u2;
    temp2 = A * temp1 + B * u1;
    x_ = temp2;
elseif tau == 3
    temp1 = A * x + B * u3;
    temp2 = A * temp1 + B * u2;
    temp3 = A * temp2 + B * u1;
    x_ = temp3;
elseif tau == 4
    temp1 = A * x + B * u4;
    temp2 = A * temp1 + B * u3;
    temp3 = A * temp2 + B * u2;
    temp4 = A * temp3 + B * u1;
    x_ = temp4;
elseif tau == 5
    temp1 = A * x + B * u5;
    temp2 = A * temp1 + B * u4;
    temp3 = A * temp2 + B * u3;
    temp4 = A * temp3 + B * u2;
    temp5 = A * temp4 + B * u1;
    x_ = temp5;
else 
    x_ = temp0;
end
y = C * x_;

== matlab function MAS_pc_up/Ps6/MATLAB Function ==
  data: x_ output size=2*1; u5 input; u4 input; u3 input; u2 input; u1 input; y output size=1*1; x input size=2*1; tau input; A input; B input; C input
function [x_,y]= fcn(u5,u4,u3,u2,u1,x,tau,A,B,C)
% tau的上界是N,最多迭代N次，控制输入按照t-s_i时刻的值
temp0 = x;
if tau == 1
    temp1 = A * x + B * u1;
    x_ = temp1;
elseif tau == 2
    temp1 = A * x + B * u2;
    temp2 = A * temp1 + B * u1;
    x_ = temp2;
elseif tau == 3
    temp1 = A * x + B * u3;
    temp2 = A * temp1 + B * u2;
    temp3 = A * temp2 + B * u1;

    x_ = temp3;
elseif tau == 4
    temp1 = A * x + B * u4;
    temp2 = A * temp1 + B * u3;
    temp3 = A * temp2 + B * u2;
    temp4 = A * temp3 + B * u1;
    x_ = temp4;
elseif tau == 5
    temp1 = A * x + B * u5;
    temp2 = A * temp1 + B * u4;
    temp3 = A * temp2 + B * u3;
    temp4 = A * temp3 + B * u2;
    temp5 = A * temp4 + B * u1;
    x_ = temp5;
else 
    x_ = temp0;
end
y = C * x_;

== matlab function MAS_pc_up/u4/MATLAB Function ==
  data: M input; y output; hat_Y input; id input
function y = fcn(M,hat_Y,id)
y = zeros(size(hat_Y(id,:)))
for i = 1:length(M(id,:))
    if M(id,i)==1
        y = y + hat_Y(i,:) - hat_Y(id,:);
    end

end

== matlab function MAS_pc_up/u5/MATLAB Function ==
  data: M input; y output; hat_Y input; id input
function y = fcn(M,hat_Y,id)
y = zeros(size(hat_Y(id,:)))
for i = 1:length(M(id,:))
    if M(id,i)==1
        y = y + hat_Y(i,:) - hat_Y(id,:)
    end

end

== matlab function MAS_pc_up/u6/MATLAB Function ==
  data: M input; y output; hat_Y input; id input
function y = fcn(M,hat_Y,id)
y = zeros(size(hat_Y(id,:)))
for i = 1:length(M(id,:))
    if M(id,i)==1
        y = y + hat_Y(i,:) - hat_Y(id,:)
    end

end

== matlab function MAS_pc_up/u_delay4/MATLAB Function ==
  data: s input; y output size=1*1; u5 input size=1*1; u4 input size=1*1; u3 input size=1*1; u2 input size=1*1; u1 input size=1*1
function y = fcn(s,u5,u4,u3,u2,u1)
if s==1
    y = u1;
elseif s==2
    y = u2;
elseif s==3
    y = u3;
elseif s==4
    y = u4;
elseif s==5
    y = u5;
else
    y = u1
disp("mmp")
end

== matlab function MAS_pc_up/u_delay5/MATLAB Function ==
  data: s input int64; y output size=1*1; u5 input size=1*1; u4 input size=1*1; u3 input size=1*1; u2 input size=1*1; u1 input size=1*1
function y = fcn(s,u5,u4,u3,u2,u1)
if s==1
    y = u1;
elseif s==2
    y = u2;
elseif s==3
    y = u3;
elseif s==4
    y = u4;
elseif s==5
    y = u5;
else 
    y = u1
disp("mmp")
end

== matlab function MAS_pc_up/u_delay6/MATLAB Function ==
  data: s input; y output size=1*1; u5 input size=1*1; u4 input size=1*1; u3 input size=1*1; u2 input size=1*1; u1 input size=1*1
function y = fcn(s,u5,u4,u3,u2,u1)
if s==1
    y = u1;
elseif s==2
    y = u2;
elseif s==3
    y = u3;
elseif s==4
    y = u4;
elseif s==5
    y = u5;
else 
    y = u1
disp("mmp3")
end

== matlab function MAS_pc_up/Ps1a2/MATLAB Function ==
  data: u10 input; u9 input; u8 input; u7 input; u6 input; x_ output size=2*1; u5 input; u4 input; u3 input; u2 input; u1 input; y output size=1*1; x input size=2*1; s input; a input; A input; B input; C input
function [x_,y]= fcn(u10,u9,u8,u7,u6,u5,u4,u3,u2,u1,x,s,a,A,B,C)
% tau的上界是N,最多迭代N次，控制输入按照t-s_i时刻的值
tau = s + a;
temp0 = x;
if tau == 1
    temp1 = A * temp0 + B * u1;
    x_ = temp1;
elseif tau == 2
    temp1 = A * temp0 + B * u2;
    temp2 = A * temp1 + B * u1;
    x_ = temp2;
elseif tau == 3
    temp1 = A * temp0 + B * u3;
    temp2 = A * temp1 + B * u2;
    temp3 = A * temp2 + B * u1;
    x_ = temp3;
elseif tau == 4
    temp1 = A * temp0 + B * u4;
    temp2 = A * temp1 + B * u3;
    temp3 = A * temp2 + B * u2;
    temp4 = A * temp3 + B * u1;
    x_ = temp4;  
elseif tau == 5
    temp1 = A * temp0 + B * u5;
    temp2 = A * temp1 + B * u4;
    temp3 = A * temp2 + B * u3;
    temp4 = A * temp3 + B * u2;
    temp5 = A * temp4 + B * u1;
    x_ = temp5;
elseif tau == 6
    temp1 = A * temp0 + B * u6;
    temp2 = A * temp1 + B * u5;
    temp3 = A * temp2 + B * u4;
    temp4 = A * temp3 + B * u3;
    temp5 = A * temp4 + B * u2;
    temp6 = A * temp5 + B * u1;
    x_ = temp6;
elseif tau == 7
    temp1 = A * temp0 + B * u7;
    temp2 = A * temp1 + B * u6;
    temp3 = A * temp2 + B * u5;
    temp4 = A * temp3 + B * u4;
    temp5 = A * temp4 + B * u3;
    temp6 = A * temp5 + B * u2;
    temp7 = A * temp6 + B * u2;
    x_ = temp7;
elseif tau == 8
    temp1 = A * temp0 + B * u8;
    temp2 = A * temp1 + B * u7;
    temp3 = A * temp2 + B * u6;
    temp4 = A * temp3 + B * u5;
    temp5 = A * temp4 + B * u4;
    temp6 = A * temp5 + B * u3;
    temp7 = A * temp6 + B * u2;
    temp8 = A * temp7 + B * u1;
    x_ = temp8;
elseif tau == 9
    temp1 = A * temp0 + B * u9;
    temp2 = A * temp1 + B * u8;
    temp3 = A * temp2 + B * u7;
    temp4 = A * temp3 + B * u6;
    temp5 = A * temp4 + B * u5;
    temp6 = A * temp5 + B * u4;
    temp7 = A * temp6 + B * u3;
    temp8 = A * temp7 + B * u2;
    temp9 = A * temp8 + B * u1;
    x_ = temp9;
elseif tau == 10
    temp1 = A * temp0 + B * u10;
    temp2 = A * temp1 + B * u9;
    temp3 = A * temp2 + B * u8;
    temp4 = A * temp3 + B * u7;
    temp5 = A * temp4 + B * u6;
    temp6 = A * temp5 + B * u5;
    temp7 = A * temp6 + B * u4;
    temp8 = A * temp7 + B * u3;
    temp9 = A * temp8 + B * u2;
    temp10 = A * temp9 + B * u1;
    x_ = temp10;
else 
    x_ = temp0;

end
y = C * x_;

== matlab function MAS_pc_up/Ps1a3/MATLAB Function ==
  data: u10 input; u9 input; u8 input; u7 input; u6 input; x_ output size=2*1; u5 input; u4 input; u3 input; u2 input; u1 input; y output size=1*1; x input size=2*1; s input; a input; A input; B input; C input
function [x_,y]= fcn(u10,u9,u8,u7,u6,u5,u4,u3,u2,u1,x,s,a,A,B,C)
% tau的上界是N,最多迭代N次，控制输入按照t-s_i时刻的值
tau = s + a;
temp0 = x;
if tau == 1
    temp1 = A * temp0 + B * u1;
    x_ = temp1;
elseif tau == 2
    temp1 = A * temp0 + B * u2;
    temp2 = A * temp1 + B * u1;
    x_ = temp2;
elseif tau == 3
    temp1 = A * temp0 + B * u3;
    temp2 = A * temp1 + B * u2;
    temp3 = A * temp2 + B * u1;
    x_ = temp3;
elseif tau == 4
    temp1 = A * temp0 + B * u4;
    temp2 = A * temp1 + B * u3;
    temp3 = A * temp2 + B * u2;
    temp4 = A * temp3 + B * u1;
    x_ = temp4;  
elseif tau == 5
    temp1 = A * temp0 + B * u5;
    temp2 = A * temp1 + B * u4;
    temp3 = A * temp2 + B * u3;
    temp4 = A * temp3 + B * u2;
    temp5 = A * temp4 + B * u1;
    x_ = temp5;
elseif tau == 6
    temp1 = A * temp0 + B * u6;
    temp2 = A * temp1 + B * u5;
    temp3 = A * temp2 + B * u4;
    temp4 = A * temp3 + B * u3;
    temp5 = A * temp4 + B * u2;
    temp6 = A * temp5 + B * u1;
    x_ = temp6;
elseif tau == 7
    temp1 = A * temp0 + B * u7;
    temp2 = A * temp1 + B * u6;
    temp3 = A * temp2 + B * u5;
    temp4 = A * temp3 + B * u4;
    temp5 = A * temp4 + B * u3;
    temp6 = A * temp5 + B * u2;
    temp7 = A * temp6 + B * u2;
    x_ = temp7;
elseif tau == 8
    temp1 = A * temp0 + B * u8;
    temp2 = A * temp1 + B * u7;
    temp3 = A * temp2 + B * u6;
    temp4 = A * temp3 + B * u5;
    temp5 = A * temp4 + B * u4;
    temp6 = A * temp5 + B * u3;
    temp7 = A * temp6 + B * u2;
    temp8 = A * temp7 + B * u1;
    x_ = temp8;
elseif tau == 9
    temp1 = A * temp0 + B * u9;
    temp2 = A * temp1 + B * u8;
    temp3 = A * temp2 + B * u7;
    temp4 = A * temp3 + B * u6;
    temp5 = A * temp4 + B * u5;
    temp6 = A * temp5 + B * u4;
    temp7 = A * temp6 + B * u3;
    temp8 = A * temp7 + B * u2;
    temp9 = A * temp8 + B * u1;
    x_ = temp9;
elseif tau == 10
    temp1 = A * temp0 + B * u10;
    temp2 = A * temp1 + B * u9;
    temp3 = A * temp2 + B * u8;
    temp4 = A * temp3 + B * u7;
    temp5 = A * temp4 + B * u6;
    temp6 = A * temp5 + B * u5;
    temp7 = A * temp6 + B * u4;
    temp8 = A * temp7 + B * u3;
    temp9 = A * temp8 + B * u2;
    temp10 = A * temp9 + B * u1;
    x_ = temp10;
else 
    x_ = temp0;

end
y = C * x_;

== matlab function MAS_pc_up/u1/MATLAB Function ==
  data: M input; y output; hat_Y input; id input
function y = fcn(M,hat_Y,id)
y = zeros(size(hat_Y(id,:)))
for i = 1:length(M(id,:))
    if M(id,i)==1
        y = y + hat_Y(i,:) - hat_Y(id,:);
    end

end
